simulink model "Intersection_Long_Lat_Gen"  (R2024b)
settings: Solver=VariableStepAuto  StartTime=0.0  StopTime=10.0  RelTol=1e-3
model workspace (MAT data in the model file):
  seed = 0
settings Model: Creator=nelsenyoung  LastModifiedBy=nelsenyoung

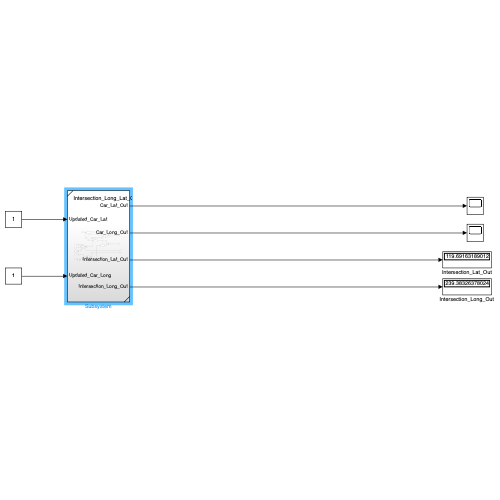
[thumbnail: Simulink's stored preview of the top-level diagram]
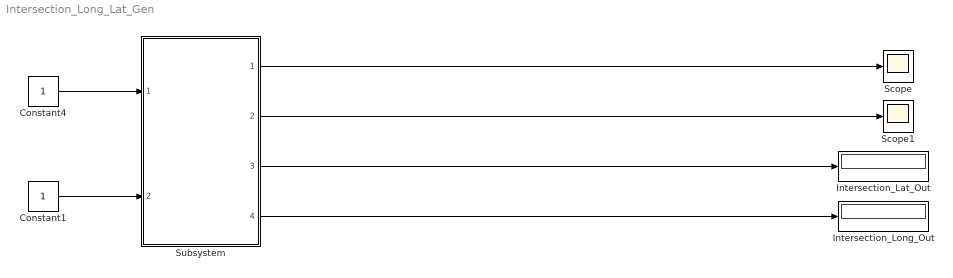
== system Intersection_Long_Lat_Gen ==
  Constant1 : Constant
  Constant4 : Constant
  Intersection_Lat_Out : Display
  Intersection_Long_Out : Display
  Scope : Scope
  Scope1 : Scope
  Subsystem : Subsystem  ReferencedSubsystem=Intersection_Long_Lat_Generator_Sub
  wires:
  Constant4/1 -> Subsystem/1
  Subsystem/1 -> Scope/1
  Subsystem/2 -> Scope1/1
  Subsystem/3 -> Intersection_Lat_Out/1
  Subsystem/4 -> Intersection_Long_Out/1
  Constant1/1 -> Subsystem/2
